simulink model "simulacionModeloMovimiento"  (R2014a)
settings: Solver=ode45  StartTime=0.0  StopTime=10.0  RelTol=1e-3
libraries: simulink x1
settings Model: Creator=PedroBarquin  LastModifiedBy=PedroBarquin

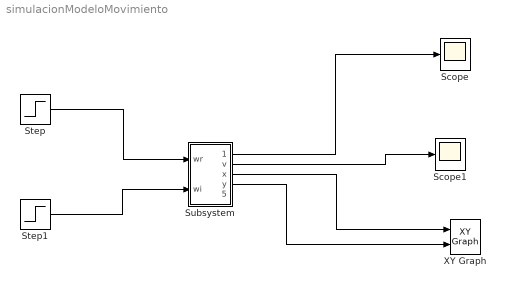
== system simulacionModeloMovimiento ==
  Scope : Scope
  Scope1 : Scope
  Step : Step  Before=1.5  After=1.5  SampleTime=0
  Step1 : Step  Before=0.5  After=0.5  SampleTime=0
  Subsystem : Subsystem  mask{r=1, L=1, x_0=1, y_0=0, theta_0=90}
  XY Graph : simulink/Sinks/XY Graph  xmin=-2  xmax=2  ymin=-2  ymax=2  st=-1
  wires:
  Step/1 -> Subsystem/1("wr ")
  Step1/1 -> Subsystem/2(wi)
  Subsystem/1("omega ") -> Scope/1
  Subsystem/2("v ") -> Scope1/1
  Subsystem/3("x ") -> XY Graph/1
  Subsystem/4("y ") -> XY Graph/2

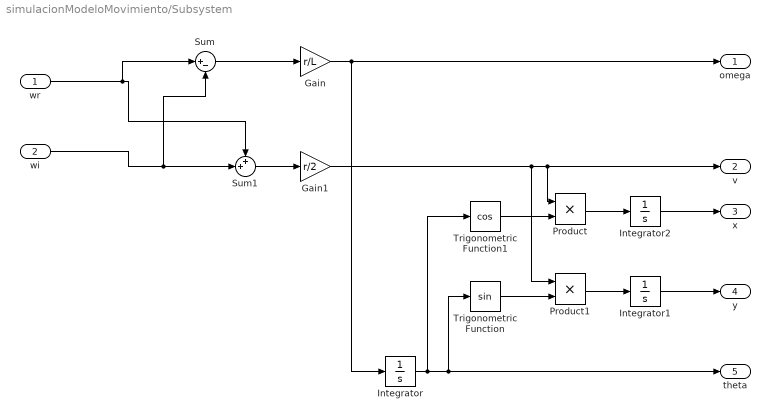
== system simulacionModeloMovimiento/Subsystem ==
  "wr " : Inport
  wi : Inport  Port=2
  Gain : Gain  Gain=r/L
  Gain1 : Gain  Gain=r/2
  Integrator : Integrator  InitialCondition=theta_0
  Integrator1 : Integrator  InitialCondition=y_0
  Integrator2 : Integrator  InitialCondition=x_0
  Product : Product
  Product1 : Product
  Sum : Sum  Inputs=|+-
  Sum1 : Sum  Inputs=++|
  Trigonometric Function : Trigonometry
  Trigonometric Function1 : Trigonometry  Operator=cos
  "omega " : Outport
  "v " : Outport  Port=2
  "x " : Outport  Port=3
  "y " : Outport  Port=4
  "theta " : Outport  Port=5
  wires:
  Gain/1 -> "omega "/1, Integrator/1
  Sum/1 -> Gain/1
  Gain1/1 -> Product1/1, "v "/1, Product/1
  Sum1/1 -> Gain1/1
  wi/1 -> Sum/2, Sum1/2
  "wr "/1 -> Sum/1, Sum1/1
  Trigonometric Function/1 -> Product1/2
  Trigonometric Function1/1 -> Product/2
  Product1/1 -> Integrator1/1
  Integrator/1 -> Trigonometric Function1/1, "theta "/1, Trigonometric Function/1
  Integrator1/1 -> "y "/1
  Product/1 -> Integrator2/1
  Integrator2/1 -> "x "/1
